simulink model "wave_test"  (R2020a)
settings: Solver=VariableStepAuto  StartTime=0.0  StopTime=2000  RelTol=1e-3
settings Model: Creator=thomas.evang  LastModifiedBy=thomas.evang

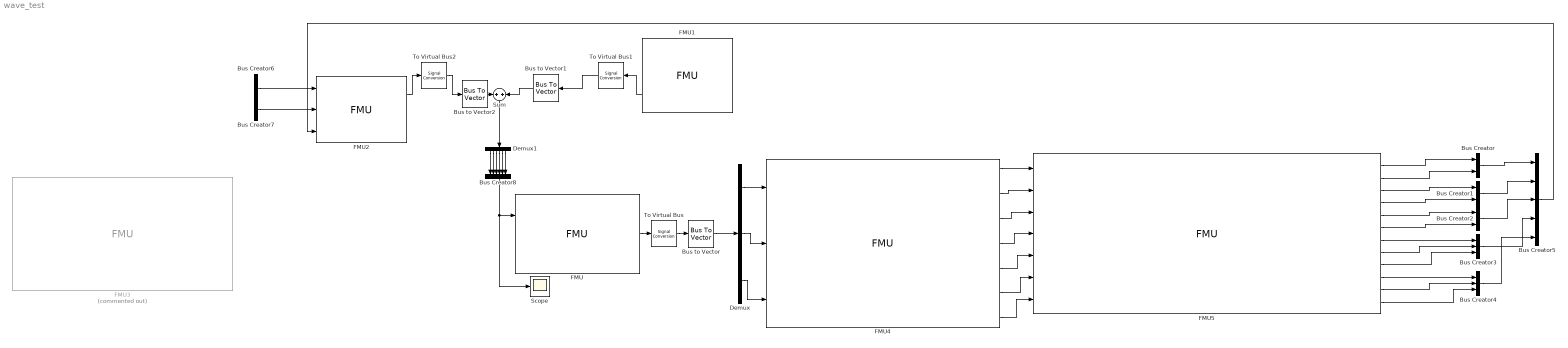
== system wave_test ==
  Bus Creator : BusCreator  Inputs=2  OutDataTypeStr=Bus: tunnel_thruster_1
      settings: InheritFromInputs=off
  Bus Creator1 : BusCreator  Inputs=2  OutDataTypeStr=Bus: tunnel_thruster_2
      settings: InheritFromInputs=off
  Bus Creator2 : BusCreator  Inputs=2  OutDataTypeStr=Bus: tunnel_thruster_3
      settings: InheritFromInputs=off
  Bus Creator3 : BusCreator  Inputs=3  OutDataTypeStr=Bus: main_propeller_port
      settings: InheritFromInputs=off
  Bus Creator4 : BusCreator  Inputs=3  OutDataTypeStr=Bus: main_propeller_starboard
      settings: InheritFromInputs=off
  Bus Creator5 : BusCreator  Inputs=5  OutDataTypeStr=Bus: thruster_states  NonVirtualBus=on
      settings: InheritFromInputs=off
  Bus Creator6 : BusCreator  Inputs=6  OutDataTypeStr=Bus: wind_forces  NonVirtualBus=on
      settings: InheritFromInputs=off
  Bus Creator7 : BusCreator  Inputs=6  OutDataTypeStr=Bus: wave_forces  NonVirtualBus=on
      settings: InheritFromInputs=off
  Bus Creator8 : BusCreator  Inputs=6  OutDataTypeStr=Bus: vessel_position  NonVirtualBus=on
      settings: InheritFromInputs=off
  Bus to Vector : BusToVector
  Bus to Vector1 : BusToVector
  Bus to Vector2 : BusToVector
  Demux : Demux  Outputs=3
  Demux1 : Demux  Outputs=6
  FMU : FMU  FMUName=dp_controller.fmu  FMUMode=CoSimulation
      mask Type: dp_controller [Co-Simulation, v2.0]
      mask Display:
      | if (exist([Simulink.fileGenControl('get','CacheFolder') '\slprj\_fmu\7923904914d3736d368090688c48e6ff\dp_controller\model.png'],'file'))
      |     image([Simulink.fileGenControl('get','CacheFolder') '\slprj\_fmu\7923904914d3736d368090688c48e6ff\dp_controller\model.png']);
      | else
      |     disp('dp_controller');
      | end
      | port_label('output',1,'force_command');
      | port_label('input',1,'vessel_position');
      | port_label('input',2,'vessel_setpoint');
  FMU1 : FMU  FMUName=linearized_wave_model.fmu  FMUMode=CoSimulation  east_drift_limit=2  k_down=1.3  k_east=2  k_north=2  k_pitch=3  k_roll=3  k_yaw=3  north_drift_limit=2  peak_frequency=0.8  wave_height=1  yaw_drift_limit=0.1745329251994329  mask(linearized_wave_model [Co-Simulation, v2.0]){}
      mask Display:
      | if (exist([Simulink.fileGenControl('get','CacheFolder') '\slprj\_fmu\e60956e6954b68356f58378614667b1c\linearized_wave_model\model.png'],'file'))
      |     image([Simulink.fileGenControl('get','CacheFolder') '\slprj\_fmu\e60956e6954b68356f58378614667b1c\linearized_wave_model\model.png']);
      | else
      |     disp('linearized_wave_model');
      | end
      | port_label('output',1,'first_order_disturbances');
      | port_label('output',2,'drift_disturbances');
  FMU2 : FMU  FMUName=vessel_model.fmu  FMUMode=CoSimulation
      mask Type: vessel_model [Co-Simulation, v2.0]
      mask Display:
      | if (exist([Simulink.fileGenControl('get','CacheFolder') '\slprj\_fmu\9625c3290247c7d7ea908bbc39a12cba\vessel_model\model.png'],'file'))
      |     image([Simulink.fileGenControl('get','CacheFolder') '\slprj\_fmu\9625c3290247c7d7ea908bbc39a12cba\vessel_model\model.png']);
      | else
      |     disp('vessel_model');
      | end
      | port_label('output',1,'ned_position');
      | port_label('output',2,'body_velocity');
      | port_label('input',1,'wind_forces');
      | port_label('input',2,'wave_forces');
      | port_label('input',3,'thruster_states');
  FMU3 : FMU  Commented=on  FMUName=dp_reference_model.fmu  FMUMode=CoSimulation  Integrator1_IC_1_=0.0  Integrator1_IC_2_=0.0  Integrator1_IC_3_=0.0  Gain1_Gain_1_=100.0  Gain1_Gain_2_=100.0  Gain1_Gain_3_=400.0  Gain3_Gain_1_=100.0  Gain3_Gain_2_=100.0  Gain3_Gain_3_=400.0  Integrator_IC_1_=0.0  Integrator_IC_2_=0.0  Integrator_IC_3_=0.0  Gain2_Gain_1_=20.0  Gain2_Gain_2_=20.0  Gain2_Gain_3_=40.0  Saturation_UpperSat_1_=1.0  Saturation_UpperSat_2_=1.0  Saturation_UpperSat_3_=0.029088820866572159  Saturation_LowerSat_1_=-1.0  Saturation_LowerSat_2_=-1.0  Saturation_LowerSat_3_=-0.029088820866572159  Saturation1_UpperSat_1_=5.0  Saturation1_UpperSat_2_=5.0  Saturation1_UpperSat_3_=1.0  Saturation1_LowerSat_1_=-5.0  Saturation1_LowerSat_2_=-5.0  Saturation1_LowerSat_3_=-1.0  mask(dp_reference_model [Co-Simulation, v2.0]){}
      mask Display:
      | if (exist([Simulink.fileGenControl('get','CacheFolder') '\slprj\_fmu\5963faaf04aaaa4d3c74431938aff70f\dp_reference_model\model.png'],'file'))
      |     image([Simulink.fileGenControl('get','CacheFolder') '\slprj\_fmu\5963faaf04aaaa4d3c74431938aff70f\dp_reference_model\model.png']);
      | else
      |     disp('dp_reference_model');
      | end
      | port_label('output',1,'filtered_setpoint.north');
      | port_label('output',2,'filtered_setpoint.east');
      | port_label('output',3,'filtered_setpoint.yaw');
      | port_label('input',1,'setpoint.north');
      | port_label('input',2,'setpoint.east');
      | port_label('input',3,'setpoint.yaw');
  FMU4 : FMU  FMUName=thrust_allocation.fmu  FMUMode=CoSimulation  Constant3_Value_1_1_=0.0  Constant3_Value_2_1_=0.0  Constant3_Value_3_1_=0.0  Constant3_Value_4_1_=0.5  Constant3_Value_5_1_=0.0  Constant3_Value_6_1_=0.5  Constant3_Value_7_1_=0.0  Constant3_Value_1_2_=0.1872  Constant3_Value_2_2_=0.1886  Constant3_Value_3_2_=0.1901  Constant3_Value_4_2_=-0.0018  Constant3_Value_5_2_=0.217  Constant3_Value_6_2_=0.0018  Constant3_Value_7_2_=0.217  Constant3_Value_1_3_=0.0058  Constant3_Value_2_3_=0.0051  Constant3_Value_3_3_=0.0045  Constant3_Value_4_3_=0.0008  Constant3_Value_5_3_=-0.0077  Constant3_Value_6_3_=-0.0008  Constant3_Value_7_3_=-0.0077  Saturation_UpperSat=144000.0  Saturation_LowerSat=-144000.0  Gain2_Gain=6.9444444444444448E-6  Gain5_Gain=100.0  Saturation1_UpperSat=144000.0  Saturation1_LowerSat=-144000.0  Gain1_Gain=6.9444444444444448E-6  Gain6_Gain=100.0  Saturation2_UpperSat=144000.0  Saturation2_LowerSat=-144000.0  Gain_Gain=6.9444444444444448E-6  Gain7_Gain=100.0  Saturation3_UpperSat=286000.0  Saturation3_LowerSat=0.0  Gain3_Gain=3.4965034965034966E-6  Gain8_Gain=100.0  Gain_Gain_c=57.295779513082323  Saturation4_UpperSat=286000.0  Saturation4_LowerSat=0.0  Gain4_Gain=3.4965034965034966E-6  Gain9_Gain=100.0  Gain_Gain_n=57.295779513082323  mask(thrust_allocation [Co-Simulation, v2.0]){}
      mask Display:
      | if (exist([Simulink.fileGenControl('get','CacheFolder') '\slprj\_fmu\474b332b791ad0f8fe35bc26f339ad5f\thrust_allocation\model.png'],'file'))
      |     image([Simulink.fileGenControl('get','CacheFolder') '\slprj\_fmu\474b332b791ad0f8fe35bc26f339ad5f\thrust_allocation\model.png']);
      | else
      |     disp('thrust_allocation');
      | end
      | port_label('output',1,'thrust_command_e.tunnel_thruster_1.rpm');
      | port_label('output',2,'thrust_command_e.tunnel_thruster_2.rpm');
      | port_label('output',3,'thrust_command_e.tunnel_thruster_3.rpm');
      | port_label('output',4,'thrust_command_e.main_propeller_port.rpm');
      | port_label('output',5,'thrust_command_e.main_propeller_port.azimuth');
      | port_label('output',6,'thrust_command_e.main_propeller_starboard.rpm');
      | port_label('output',7,'thrust_command_e.main_propeller_starboard.azimuth');
      | port_label('input',1,'force_command.surge');
      | port_label('input',2,'force_command.sway');
      | port_label('input',3,'force_command.yaw');
  FMU5 : FMU  FMUName=thruster_model.fmu  FMUMode=CoSimulation
      mask Type: thruster_model [Co-Simulation, v2.0]
      mask Display:
      | if (exist([Simulink.fileGenControl('get','CacheFolder') '\slprj\_fmu\16b631dc9d41cba3577a5daa9855a37f\thruster_model\model.png'],'file'))
      |     image([Simulink.fileGenControl('get','CacheFolder') '\slprj\_fmu\16b631dc9d41cba3577a5daa9855a37f\thruster_model\model.png']);
      | else
      |     disp('thruster_model');
      | end
      | port_label('output',1,'thruster_states_i.tunnel_thruster_1.power_consumption');
      | port_label('output',2,'thruster_states_i.tunnel_thruster_1.thrust');
      | port_label('output',3,'thruster_states_i.tunnel_thruster_2.power_consumption');
      | port_label('output',4,'thruster_states_i.tunnel_thruster_2.thrust');
      | port_label('output',5,'thruster_states_i.tunnel_thruster_3.power_consumption');
      | port_label('output',6,'thruster_states_i.tunnel_thruster_3.thrust');
      | port_label('output',7,'thruster_states_i.main_propeller_port.power_consumption');
      | port_label('output',8,'thruster_states_i.main_propeller_port.thrust');
      | port_label('output',9,'thruster_states_i.main_propeller_port.azimuth');
      | port_label('output',10,'thruster_states_i.main_propeller_starboard.power_consumption');
      | port_label('output',11,'thruster_states_i.main_propeller_starboard.thrust');
      | port_label('output',12,'thruster_states_i.main_propeller_starboard.azimuth');
      | port_label('input',1,'thrust_command_n.tunnel_thruster_1.rpm');
      | port_label('input',2,'thrust_command_n.tunnel_thruster_2.rpm');
      | port_label('input',3,'thrust_command_n.tunnel_thruster_3.rpm');
      | port_label('input',4,'thrust_command_n.main_propeller_port.rpm');
      | port_label('input',5,'thrust_command_n.main_propeller_port.azimuth');
      | port_label('input',6,'thrust_command_n.main_propeller_starboard.rpm');
      | port_label('input',7,'thrust_command_n.main_propeller_starboard.azimuth');
  Scope : Scope
  Sum : Sum  Inputs=+|+
  To Virtual Bus : SignalConversion  ConversionOutput=Virtual bus  OverrideOpt=off
  To Virtual Bus1 : SignalConversion  ConversionOutput=Virtual bus  OverrideOpt=off
  To Virtual Bus2 : SignalConversion  ConversionOutput=Virtual bus  OverrideOpt=off
  wires:
  FMU1/2 -> To Virtual Bus1/1
  Demux/1 -> FMU4/1
  Demux/2 -> FMU4/2
  Demux/3 -> FMU4/3
  FMU4/1 -> FMU5/1
  FMU4/2 -> FMU5/2
  FMU4/3 -> FMU5/3
  FMU4/4 -> FMU5/4
  FMU4/5 -> FMU5/5
  FMU4/6 -> FMU5/6
  FMU4/7 -> FMU5/7
  FMU5/1 -> Bus Creator/1
  FMU5/2 -> Bus Creator/2
  FMU5/3 -> Bus Creator1/1
  FMU5/4 -> Bus Creator1/2
  FMU5/5 -> Bus Creator2/1
  FMU5/6 -> Bus Creator2/2
  FMU5/7 -> Bus Creator3/1
  FMU5/8 -> Bus Creator3/2
  FMU5/9 -> Bus Creator3/3
  FMU5/10 -> Bus Creator4/1
  FMU5/12 -> Bus Creator4/3
  FMU5/11 -> Bus Creator4/2
  Bus Creator/1 -> Bus Creator5/1
  Bus Creator1/1 -> Bus Creator5/2
  Bus Creator2/1 -> Bus Creator5/3
  Bus Creator3/1 -> Bus Creator5/4
  Bus Creator4/1 -> Bus Creator5/5
  Bus Creator5/1 -> FMU2/3
  FMU/1 -> To Virtual Bus/1
  To Virtual Bus/1 -> Bus to Vector/1
  Bus to Vector/1 -> Demux/1
  Bus Creator6/1 -> FMU2/1
  Bus Creator7/1 -> FMU2/2
  Demux1/1 -> Bus Creator8/1
  Demux1/2 -> Bus Creator8/2
  Demux1/3 -> Bus Creator8/3
  Demux1/4 -> Bus Creator8/4
  Demux1/5 -> Bus Creator8/5
  Demux1/6 -> Bus Creator8/6
  Bus Creator8/1 -> Scope/1, FMU/1
  Sum/1 -> Demux1/1
  Bus to Vector1/1 -> Sum/2
  Bus to Vector2/1 -> Sum/1
  To Virtual Bus1/1 -> Bus to Vector1/1
  FMU2/1 -> To Virtual Bus2/1
  To Virtual Bus2/1 -> Bus to Vector2/1
